simulink model "BD_HESS_K"  (R2024b)
settings: Solver=ode1  StartTime=0.0  StopTime=1369  FixedStep=0.1  MaxStep=1  RelTol=1e-3  AbsTol=1e-3
values from neighbouring files (symbols this model uses):
  ess2_cap = [ ... (first row only)    [ESS2_SC_MaxwellBCAP3400F.m]
  ess2_cap_scale = 1    [ESS2_SC_MaxwellBCAP3400F.m]
  ess2_coulombic_eff = [ ... (first row only)    [ESS2_SC_MaxwellBCAP3400F.m]
  ess2_init_soc = 1    [ESS2_SC_MaxwellBCAP3400F.m]
  ess2_max_volts = 2.7*120    (= 324)    [ESS2_SC_MaxwellBCAP3400F.m]
  ess2_min_volts = 0*2.7*120    (= 0)    [ESS2_SC_MaxwellBCAP3400F.m]
  ess2_mod_init_tmp = 20    [ESS2_SC_MaxwellBCAP3400F.m]
  ess2_module_num = 1    [ESS2_SC_MaxwellBCAP3400F.m]
  ess2_parallel_mod_num = 1    [ESS2_SC_MaxwellBCAP3400F.m]
  ess2_r = [ ... (first row only)    [ESS2_SC_MaxwellBCAP3400F.m]
  ess2_res_scale_coef = [1 0 1 0]    [ESS2_SC_MaxwellBCAP3400F.m]
  ess2_res_scale_fun = inline('(x(1)*ess2_module_num+x(2))/(x(3)*ess2_cap_scale+x(4))','x','ess2_module_num','ess2_cap_scale')    [ESS2_SC_MaxwellBCAP3400F.m]
  ess2_tmp = [-20 -10 0 5 10 15 20 25 30 40 50 60 65]    [ESS2_SC_MaxwellBCAP3400F.m]
  ess_cap_scale = 1    [ESS_Panasonic_NCR18650B_params.m]
  ess_coulombic_eff = [0.863 0.957 0.959 0.967 0.994]    [ESS_Panasonic_NCR18650B_params.m]
  ess_init_soc = 1    [ESS_Panasonic_NCR18650B_params.m]
  ess_max_ah_cap = [2.78 2.92 3.09 3.27 3.31]*74    [ESS_Panasonic_NCR18650B_params.m]
  ess_max_volts = 4.2*6    (= 25.2)    [ESS_Panasonic_NCR18650B_params.m]
  ess_min_volts = 2.5*6    (= 15)    [ESS_Panasonic_NCR18650B_params.m]
  ess_mod_init_tmp = 20    [ESS_Panasonic_NCR18650B_params.m]
  ess_module_num = 16    [ESS_Panasonic_NCR18650B_params.m]
  ess_on = 1    [ESS_Panasonic_NCR18650B_params.m]
  ess_r_chg = [0.0470 0.0457 0.0448 0.0435 0.0429 0.0427 0.0429 0.0462 ... (first row only)    [ESS_Panasonic_NCR18650B_params.m]
  ess_r_dis = [0.0470 0.0457 0.0448 0.0435 0.0429 0.0427 0.0429 0.0462 ... (first row only)    [ESS_Panasonic_NCR18650B_params.m]
  ess_res_scale_coef = [1 0 1 0]    [ESS_Panasonic_NCR18650B_params.m]
  ess_res_scale_fun = inline('(x(1)*ess_module_num+x(2))/(x(3)*ess_cap_scale+x(4))','x','ess_module_num','ess_cap_scale')    [ESS_Panasonic_NCR18650B_params.m]
  ess_soc = [0 10 20 40 60 80 90 100]/100    [ESS_Panasonic_NCR18650B_params.m]
  ess_tmp = [-10 0 10 25 45]    [ESS_Panasonic_NCR18650B_params.m]
  ess_voc = [2.5 2.74 2.93 3.17 3.36 3.5 3.49 3.34 ... (first row only)    [ESS_Panasonic_NCR18650B_params.m]
  mc_min_volts = 0    [ESS_Panasonic_NCR18650B_params.m]
  pth = pth_values(i)    [Ems_code_for_set_EMSvalue.m]
undefined symbols (not defined in the file or in its folder): power_load_in_Watt
(part 2 of 2)

== system BD_HESS_K/battery pack <ess>/pack Voc, Rint ==
  SOC (prev) : Inport
  req'd battery power (W) : Inport  Port=2
  mod tmp (C) : Inport  Port=3
  #bty : Constant  Value=ess_module_num
  Product : Product  InputSameDT=on  RndMeth=Zero  SaturateOnIntegerOverflow=on  OutDataTypeStr=Inherit: Same as first input
  Rchg (ohms) : Subsystem  mask(2-D Table Lookup){xindex=ess_tmp, yindex=ess_soc, table=ess_r_chg}
      mask prompts: xindex "X Index"; yindex "Y Index"
      mask help:
      | Two Dimensional Table Lookup
      | The first input corresponds to X Index and the second input corresponds to the Y Index
      mask init:
      | sftab2chk(xindex,yindex,table);
      mask Help: This block returns a linearly interpolated intersection from the table using the X index (which corresponds to the rows of the table) and the Y index (which corresponds to the columns of the table).  Extrapolation is used.
      mask Display: plot(-10,-10,110,110,[90,50,10],[90,40,30],[90,50,10],[50,26,20],[90,50,10],[22,13,10])
  Rdis (ohms) : Subsystem  mask(2-D Table Lookup){xindex=ess_tmp, yindex=ess_soc, table=ess_r_dis}
      mask prompts: xindex "X Index"; yindex "Y Index"
      mask help:
      | Two Dimensional Table Lookup
      | The first input corresponds to X Index and the second input corresponds to the Y Index
      mask init:
      | sftab2chk(xindex,yindex,table);
      mask Help: This block returns a linearly interpolated intersection from the table using the X index (which corresponds to the rows of the table) and the Y index (which corresponds to the columns of the table).  Extrapolation is used.
      mask Display: plot(-10,-10,110,110,[90,50,10],[90,40,30],[90,50,10],[50,26,20],[90,50,10],[22,13,10])
  Switch : Switch
  VOC (V) : Subsystem  mask(2-D Table Lookup){xindex=ess_tmp, yindex=ess_soc, table=ess_voc}
      mask prompts: xindex "X Index"; yindex "Y Index"
      mask help:
      | Two Dimensional Table Lookup
      | The first input corresponds to X Index and the second input corresponds to the Y Index
      mask init:
      | sftab2chk(xindex,yindex,table);
      mask Help: This block returns a linearly interpolated intersection from the table using the X index (which corresponds to the rows of the table) and the Y index (which corresponds to the columns of the table).  Extrapolation is used.
      mask Display: plot(-10,-10,110,110,[90,50,10],[90,40,30],[90,50,10],[50,26,20],[90,50,10],[22,13,10])
  resistance scale fun : Gain  Gain=ess_res_scale_fun(ess_res_scale_coef,ess_module_num,ess_cap_scale)  SaturateOnIntegerOverflow=on  OutDataTypeStr=Inherit: Same as input  ParamDataTypeStr=Inherit: Same as input
  resistance scale fun1 : Gain  Gain=ess_res_scale_fun(ess_res_scale_coef,ess_module_num,ess_cap_scale)  SaturateOnIntegerOverflow=on  OutDataTypeStr=Inherit: Same as input  ParamDataTypeStr=Inherit: Same as input
  pack open- circuit voltage : Outport  InitialOutput=0
  pack resistance : Outport  Port=2  InitialOutput=0
  wires:
  resistance scale fun1/1 -> Switch/3
  Rchg (ohms)/1(table out) -> resistance scale fun1/1
  resistance scale fun/1 -> Switch/1
  Rdis (ohms)/1(table out) -> resistance scale fun/1
  Switch/1 -> pack resistance/1
  #bty/1 -> Product/2
  Product/1 -> pack open- circuit voltage/1
  VOC (V)/1(table out) -> Product/1
  req'd battery power (W)/1 -> Switch/2
  SOC (prev)/1 -> VOC (V)/2(y0), Rdis (ohms)/2(y0), Rchg (ohms)/2(y0)
  mod tmp (C)/1 -> VOC (V)/1(x0), Rdis (ohms)/1(x0), Rchg (ohms)/1(x0)

== system BD_HESS_K/battery pack <ess>/stop sim ==
  SOC : Inport
  Enable : EnablePort
  Const : Constant  Value=.001
  Relational Operator : RelationalOperator  Operator=<
  Stop Simulation : Stop
  wires:
  Const/1 -> Relational Operator/2
  SOC/1 -> Relational Operator/1
  Relational Operator/1 -> Stop Simulation/1

== system BD_HESS_K/SC pack <ess2> /Calc Iout/SOC limit ==
  SOC : Inport
  Pbty : Inport  Port=2
  Constant1 : Constant  Value=0.001
  Constant5 : Constant  Value=.999
  Constant9 : Constant  Value=0
  Logical Operator : Logic  Operator=OR
  Logical Operator1 : Logic
  Logical Operator2 : Logic  Operator=NOT  Inputs=1
  Relational Operator : RelationalOperator  Operator=>
  Relational Operator3 : RelationalOperator  Operator=<
  SOC>=.999 : RelationalOperator
  charging (Preq is neg) : RelationalOperator  Operator=<
  no power req if SOC<0 and trying to discharge : Switch  Threshold=eps
  no power req if SOC>.999 and trying to charge : Switch  Threshold=eps
  "Pbty, limited" : Outport  InitialOutput=0
  tag scope: ess2_soc_hi_limited=global, ess2_soc_low_limited=global
  wires:
  Constant1/1 -> Relational Operator/2
  Pbty/1 -> Relational Operator3/1, charging (Preq is neg)/1, no power req if SOC<0 and trying to discharge/1
  Logical Operator/1 -> Logical Operator2/1, no power req if SOC<0 and trying to discharge/2
  SOC/1 -> Relational Operator/1, SOC>=.999/1
  SOC>=.999/1 -> Logical Operator1/1
  charging (Preq is neg)/1 -> Logical Operator1/2
  Constant5/1 -> SOC>=.999/2
  no power req if SOC<0 and trying to discharge/1 -> no power req if SOC>.999 and trying to charge/3
  no power req if SOC>.999 and trying to charge/1 -> "Pbty, limited"/1
  Logical Operator1/1 -> [ess2_soc_hi_limited], no power req if SOC>.999 and trying to charge/2
  Relational Operator3/1 -> Logical Operator/2
  Constant9/1 -> no power req if SOC<0 and trying to discharge/3, no power req if SOC>.999 and trying to charge/1, Relational Operator3/2, charging (Preq is neg)/2
  Relational Operator/1 -> Logical Operator/1
  Logical Operator2/1 -> [ess2_soc_low_limited]

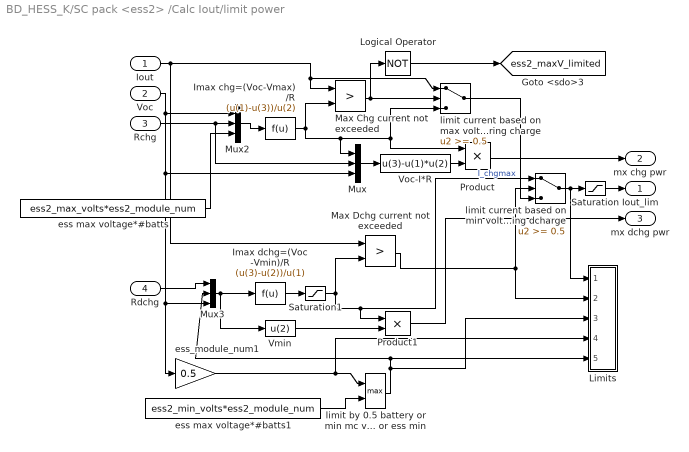
== system BD_HESS_K/SC pack <ess2> /Calc Iout/limit power ==
  Iout : Inport
  Voc : Inport  Port=2
  Rchg : Inport  Port=3
  Rdchg : Inport  Port=4
  Imax chg=(Voc-Vmax)/R : Fcn  Expr=(u(1)-u(3))/u(2)
  Imax dchg=(Voc -Vmin)/R : Fcn  Expr=(u(3)-u(2))/u(1)
  Limits : Subsystem
  Logical Operator : Logic  Operator=NOT
  Max Chg current not exceeded : RelationalOperator  Operator=>
  Max Dchg current not exceeded : RelationalOperator  Operator=>
  Mux : Mux  Inputs=3
  Mux2 : Mux  Inputs=3
  Mux3 : Mux  Inputs=3
  Product : Product  InputSameDT=on  RndMeth=Zero  SaturateOnIntegerOverflow=on  OutDataTypeStr=Inherit: Same as first input
  Product1 : Product  InputSameDT=on  RndMeth=Zero  SaturateOnIntegerOverflow=on  OutDataTypeStr=Inherit: Same as first input
  Saturation : Saturate  UpperLimit=2600*ess2_parallel_mod_num  LowerLimit=-2600*ess2_parallel_mod_num
  Saturation1 : Saturate  UpperLimit=inf  LowerLimit=0
  Vmin : Fcn  Expr=u(2)
  Voc-I*R : Fcn  Expr=u(3)-u(1)*u(2)
  ess max voltage*#batts : Constant  Value=ess2_max_volts*ess2_module_num
  ess max voltage*#batts1 : Constant  Value=ess2_min_volts*ess2_module_num
  ess_module_num1 : Gain  Gain=0.5  SaturateOnIntegerOverflow=on  OutDataTypeStr=Inherit: Same as input  ParamDataTypeStr=Inherit: Same as input
  limit by 0.5 battery or min mc voltage or ess min : MinMax  Function=max  Inputs=2  InputSameDT=on  SaturateOnIntegerOverflow=on
  limit current based on max voltage during charge : Switch  Threshold=0.5
  limit current based on min voltage during dcharge : Switch  Threshold=0.5
  Iout_lim : Outport
  mx chg pwr : Outport  Port=2
  mx dchg pwr : Outport  Port=3
  tag scope: ess2_maxV_limited=global
  wires:
  Mux2/1 -> Imax chg=(Voc-Vmax)/R/1
  Iout/1 -> Max Chg current not exceeded/1, limit current based on max voltage during charge/1, Max Dchg current not exceeded/1
  Imax chg=(Voc-Vmax)/R/1 -> Max Chg current not exceeded/2, Mux/1, limit current based on max voltage during charge/3, Product/1
  Rchg/1 -> Mux2/2, Mux/2
  Voc/1 -> Mux2/1, Mux/3, Mux3/3, ess_module_num1/1
  Mux/1 -> Voc-I*R/1
  Voc-I*R/1 -> Product/2
  Product/1 -> mx chg pwr/1
  Max Chg current not exceeded/1 -> limit current based on max voltage during charge/2, Logical Operator/1
  Logical Operator/1 -> [ess2_maxV_limited]
  ess max voltage*#batts/1 -> Mux2/3
  limit current based on max voltage during charge/1 -> limit current based on min voltage during dcharge/3  "I_chgmax"
  limit current based on min voltage during dcharge/1 -> Saturation/1, Limits/1(current req)
  Mux3/1 -> Imax dchg=(Voc -Vmin)/R/1, Vmin/1
  Imax dchg=(Voc -Vmin)/R/1 -> Saturation1/1
  Rdchg/1 -> Mux3/1
  Max Dchg current not exceeded/1 -> limit current based on min voltage during dcharge/2, Limits/2(current bat limited)
  ess max voltage*#batts1/1 -> limit by 0.5 battery or min mc voltage or ess min/2
  ess_module_num1/1 -> limit by 0.5 battery or min mc voltage or ess min/1, Limits/4(V battery (.5Voc))
  limit by 0.5 battery or min mc voltage or ess min/1 -> Limits/3(V used), Mux3/2, Limits/5(V ess_min_volts)
  Vmin/1 -> Product1/2
  Product1/1 -> mx dchg pwr/1
  Saturation/1 -> Iout_lim/1
  Saturation1/1 -> Max Dchg current not exceeded/2, Product1/1, limit current based on min voltage during dcharge/1

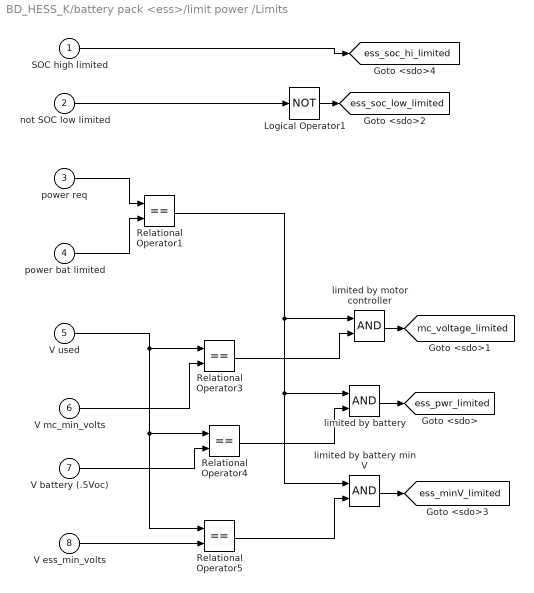
== system BD_HESS_K/battery pack <ess>/limit power /Limits ==
  SOC high limited : Inport
  not SOC low limited : Inport  Port=2
  power req : Inport  Port=3
  power bat limited : Inport  Port=4
  V used : Inport  Port=5
  V mc_min_volts : Inport  Port=6
  V battery (.5Voc) : Inport  Port=7
  V ess_min_volts : Inport  Port=8
  Logical Operator1 : Logic  Operator=NOT  Inputs=1
  Relational Operator{1,3..5} (4 alike) : RelationalOperator  Operator===
  limited by battery : Logic
  limited by battery min V : Logic
  limited by motor controller : Logic
  tag scope: ess_minV_limited=global, ess_pwr_limited=global, ess_soc_hi_limited=global, ess_soc_low_limited=global, mc_voltage_limited=global
  wires:
  power bat limited/1 -> Relational Operator1/2
  V mc_min_volts/1 -> Relational Operator3/2
  V used/1 -> Relational Operator3/1, Relational Operator4/1, Relational Operator5/1
  V battery (.5Voc)/1 -> Relational Operator4/2
  V ess_min_volts/1 -> Relational Operator5/2
  limited by motor controller/1 -> [mc_voltage_limited]
  limited by battery/1 -> [ess_pwr_limited]
  limited by battery min V/1 -> [ess_minV_limited]
  Relational Operator3/1 -> limited by motor controller/2
  Relational Operator1/1 -> limited by motor controller/1, limited by battery/1, limited by battery min V/1
  Relational Operator4/1 -> limited by battery/2
  Relational Operator5/1 -> limited by battery min V/2
  power req/1 -> Relational Operator1/1
  Logical Operator1/1 -> [ess_soc_low_limited]
  not SOC low limited/1 -> Logical Operator1/1
  SOC high limited/1 -> [ess_soc_hi_limited]

== system BD_HESS_K/battery pack <ess>/max pack pwr (W)1/Rchg (ohms)1 ==
  x0 : Inport
  y0 : Inport  Port=2
  Mux : Mux  Inputs=2
  S-function : S-Function  FunctionName=sftable2  Parameters=xindex, yindex, table  SFunctionDeploymentMode=off  EnableBusSupport=off
  table out : Outport  InitialOutput=0
  wires:
  Mux/1 -> S-function/1
  x0/1 -> Mux/1
  S-function/1 -> table out/1
  y0/1 -> Mux/2

== system BD_HESS_K/battery pack <ess>/max pack pwr (W)1/Rdis (ohms) ==
  x0 : Inport
  y0 : Inport  Port=2
  Mux : Mux  Inputs=2
  S-function : S-Function  FunctionName=sftable2  Parameters=xindex, yindex, table  SFunctionDeploymentMode=off  EnableBusSupport=off
  table out : Outport  InitialOutput=0
  wires:
  Mux/1 -> S-function/1
  x0/1 -> Mux/1
  S-function/1 -> table out/1
  y0/1 -> Mux/2

== system BD_HESS_K/battery pack <ess>/max pack pwr (W)1/VOC (V) ==
  x0 : Inport
  y0 : Inport  Port=2
  Mux : Mux  Inputs=2
  S-function : S-Function  FunctionName=sftable2  Parameters=xindex, yindex, table  SFunctionDeploymentMode=off  EnableBusSupport=off
  table out : Outport  InitialOutput=0
  wires:
  Mux/1 -> S-function/1
  x0/1 -> Mux/1
  S-function/1 -> table out/1
  y0/1 -> Mux/2

== system BD_HESS_K/battery pack <ess>/pack Voc, Rint/Rchg (ohms) ==
  x0 : Inport
  y0 : Inport  Port=2
  Mux : Mux  Inputs=2
  S-function : S-Function  FunctionName=sftable2  Parameters=xindex, yindex, table  SFunctionDeploymentMode=off  EnableBusSupport=off
  table out : Outport  InitialOutput=0
  wires:
  y0/1 -> Mux/2
  S-function/1 -> table out/1
  x0/1 -> Mux/1
  Mux/1 -> S-function/1

== system BD_HESS_K/battery pack <ess>/pack Voc, Rint/Rdis (ohms) ==
  x0 : Inport
  y0 : Inport  Port=2
  Mux : Mux  Inputs=2
  S-function : S-Function  FunctionName=sftable2  Parameters=xindex, yindex, table  SFunctionDeploymentMode=off  EnableBusSupport=off
  table out : Outport  InitialOutput=0
  wires:
  y0/1 -> Mux/2
  S-function/1 -> table out/1
  x0/1 -> Mux/1
  Mux/1 -> S-function/1

== system BD_HESS_K/battery pack <ess>/pack Voc, Rint/VOC (V) ==
  x0 : Inport
  y0 : Inport  Port=2
  Mux : Mux  Inputs=2
  S-function : S-Function  FunctionName=sftable2  Parameters=xindex, yindex, table  SFunctionDeploymentMode=off  EnableBusSupport=off
  table out : Outport  InitialOutput=0
  wires:
  y0/1 -> Mux/2
  S-function/1 -> table out/1
  x0/1 -> Mux/1
  Mux/1 -> S-function/1

== system BD_HESS_K/SC pack <ess2> /Calc Iout/limit power/Limits ==
  current req : Inport
  current bat limited : Inport  Port=2
  V used : Inport  Port=3
  V battery (.5Voc) : Inport  Port=4
  V ess_min_volts : Inport  Port=5
  Relational Operator1 : RelationalOperator  Operator===
  Relational Operator4 : RelationalOperator  Operator===
  Relational Operator5 : RelationalOperator  Operator=<=
  limited by battery : Logic
  limited by battery min V : Logic
  tag scope: ess2_minV_limited=global, ess2_pwr_limited=global
  wires:
  current bat limited/1 -> Relational Operator1/2
  V used/1 -> Relational Operator4/1, Relational Operator5/1
  V battery (.5Voc)/1 -> Relational Operator4/2
  V ess_min_volts/1 -> Relational Operator5/2
  limited by battery/1 -> [ess2_pwr_limited]
  limited by battery min V/1 -> [ess2_minV_limited]
  Relational Operator1/1 -> limited by battery/1, limited by battery min V/1
  Relational Operator4/1 -> limited by battery/2
  Relational Operator5/1 -> limited by battery min V/2
  current req/1 -> Relational Operator1/1
